simulink model "PID_cascaded_control"  (R2025a)
settings: Solver=FixedStepAuto  StartTime=0.0  StopTime=60  FixedStep=0.01  RelTol=1e-3
InitFcn:
  | parameters
values from neighbouring files (symbols this model uses):
  A = pi*(d/2)^2    (= 0.00321699087728)    [parameters.m]    (also in simulations_code.m = 0.00785398163397; test.m = 0.00785398163397)
  A_cross = 0.090    (= 0.09)    [parameters.m]    (also in simulations_code.m = 0.07; test.m = 0.07)
  C_d = 0.136    [parameters.m]    (also in simulations_code.m = 1; test.m = 1)
  constant_amplitude = 0    [Mission.m]    (also in sensitivity.m)
  d1 = 2    [parameters.m]    (also in simulation_matlab.m = 5; simulations_code.m = 5; test.m = 5)
  disturbance_start_time = 120    [compare_controllers.m]    (also in sensitivity.m = 0)
  F_pos = 0.300 * g + m*g    (= 49.70727)    [parameters.m]    (also in sensitivity.m = 0.300 * g + m_values(i)*g; simulation_matlab.m = 2.94; simulations_code.m = 32.37; test.m = 32.37)
  g = 9.81    [parameters.m]    (also in simulation_matlab.m; simulations_code.m; test.m)
  I_hold = 0    [parameters.m]
  I_move = 1.5    [parameters.m]
  m = 4.567+0.2    (= 4.767)    [parameters.m]    (also in simulation_matlab.m = 3; simulations_code.m = 3; test.m = 3)
  m_a = 0    [parameters.m]    (also in simulation_matlab.m; simulations_code.m = 2.5; test.m = 2.5)
  p = 0.002    [parameters.m]    (also in simulation_matlab.m; simulations_code.m; test.m)
  rho = 1000    [parameters.m]    (also in simulation_matlab.m; simulations_code.m; test.m)
  rpm_max = 150    [parameters.m]
  sine_amplitude = 0    [Mission.m]    (also in sensitivity.m)
  sine_frequency = 0.05    [Mission.m]    (also in sensitivity.m)
  V_supply = 11.1    [parameters.m]
  x_max = V_max / A    (= 0.155424749113)    [parameters.m]    (also in simulations_code.m = 0.0636619772368)
libraries: slpidlib x2
settings Model: Creator=hannasennero  LastModifiedBy=hannasennero
settings SolverCC: ZeroCrossAlgorithm=Adaptive
settings DebuggingCC: IgnoredZcDiagnostic=none

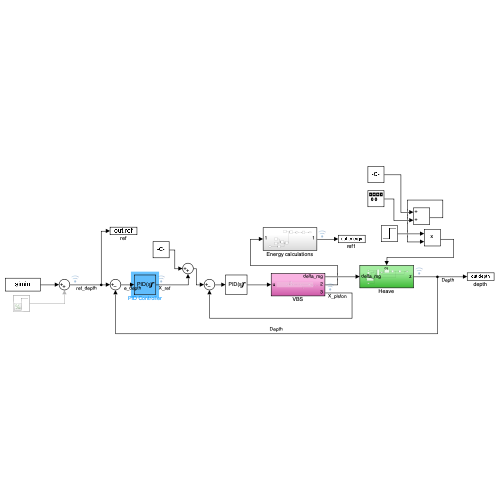
[thumbnail: Simulink's stored preview of the top-level diagram]
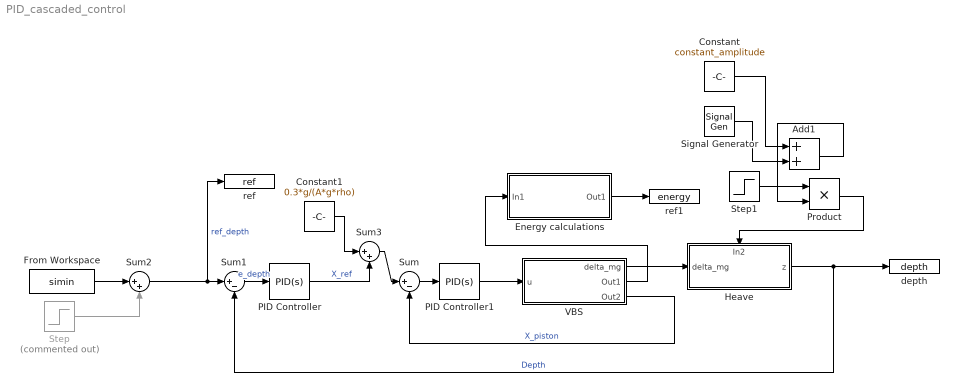
== system PID_cascaded_control ==
  Add1 : Sum
  Constant : Constant  Value=constant_amplitude
  Constant1 : Constant  Value=0.3*g/(A*g*rho)
  Energy calculations : Subsystem
  From Workspace : FromWorkspace  VariableName=simin
  Heave : Subsystem
      settings: PortSchema="{\"entries\":[{\"content\":{\"sides\":[{\"content\":{\"connectorIds\":[\"In1\"]},\"type\":\"ConnectorPlacement.EquallySpacedRectSide\",\"uuid\":\"6f6a1a60-77e6-4781-930b-afddbe975a8d\"},{\"content\":{\"connectorIds\":[\"Out1\"],\"side\":\"RIGHT\"},\"type\":\"ConnectorPlacement.EquallySpacedRectSide\",\"uuid\":\"4976a1b4-b4d2-4f2a-94be-bdc8db839add\"},{\"content\":{\"connectorIds\":[\"In2\"],\"side\":\"TOP\"},\"type\":\"ConnectorPlacement.EquallySpacedRectSide\",\"uuid\":\"504c6e21-38d1-42a8-8b7b-eda0c51b3613\"}]},\"type\":\"ConnectorPlacement.EquallySpacedConnector\",\"uuid\":\"116e8cad-2b5c-4ef7-8338-d893e08918e3\"}],\"packageUris\":[\"http://schema.mathworks.com/mf0/Connector/R2020b\"],\"version\":\"1.0\"}"
  PID Controller : slpidlib/PID Controller  Controller=PID  Form=Parallel  TimeDomain=Continuous-time  UseExternalTs=off  SampleTime=-1  IntegratorMethod=Forward Euler  FilterMethod=Forward Euler  ControllerParametersSource=internal  P=0.1  I=0  UseKiTs=off  D=2  UseExternalDerivativeSource=off  N=10  UseFilter=on  TunerSelectOption=Transfer Function Based (PID Tuner App)  InitialConditionSource=internal  InitialConditionForIntegrator=0  InitialConditionForFilter=0  DifferentiatorICPrevScaledInput=0  ExternalReset=none  TrackingMode=off  Kt=1  LimitOutput=on  SatLimitsSource=internal  UpperSaturationLimit=x_max-0.0003/A  LowerSaturationLimit=-0.0003/A  LinearizeAsGain=off  AntiWindupMode=none  Kb=1  LimitIntegrator=off  UpperIntegratorSaturationLimit=inf  LowerIntegratorSaturationLimit=-inf  POutMin=[]  POutMax=[]  IOutMin=[]  IOutMax=[]  DOutMin=[]  DOutMax=[]  NOutMin=[]  NOutMax=[]  SumOutMin=[]  SumOutMax=[]  SaturationOutMin=[]  SaturationOutMax=[]  PParamMin=[]  PParamMax=[]  IParamMin=[]  IParamMax=[]  DParamMin=[]  DParamMax=[]  NParamMin=[]  NParamMax=[]  KbParamMin=[]  KbParamMax=[]  KtParamMin=[]  KtParamMax=[]  KbOutMin=[]  KbOutMax=[]  KtOutMin=[]  KtOutMax=[]  IntegratorOutMin=[]  IntegratorOutMax=[]  FilterOutMin=[]  FilterOutMax=[]  SumI1OutMin=[]  SumI1OutMax=[]  SumI2OutMin=[]  SumI2OutMax=[]  SumI3OutMin=[]  SumI3OutMax=[]  SumI4OutMin=[]  SumI4OutMax=[]  SumDOutMin=[]  SumDOutMax=[]  DifferentiatorOutMin=[]  DifferentiatorOutMax=[]  FilterDiffOutCoefMin=[]  FilterDiffOutCoefMax=[]  ReciprocalOutMin=[]  ReciprocalOutMax=[]  SumDenOutMin=[]  SumDenOutMax=[]  SumNumOutMin=[]  SumNumOutMax=[]  DivideOutMin=[]  DivideOutMax=[]  UdiffTsProdOutMin=[]  UdiffTsProdOutMax=[]  NTsProdOutMin=[]  NTsProdOutMax=[]  UintegralTsProdOutMin=[]  UintegralTsProdOutMax=[]  UngainTsProdOutMin=[]  UngainTsProdOutMax=[]  ClampingZeroOutDataTypeStr=Inherit: Inherit via back propagation  ClampingZeroOutMin=[]  ClampingZeroOutMax=[]  FilterDenConstantOutDataTypeStr=Inherit: Inherit via back propagation  FilterDenConstantOutMin=[]  FilterDenConstantOutMax=[]  PCopyOutDataTypeStr=Inherit: Inherit via back propagation  PCopyOutMin=[]  PCopyOutMax=[]  NCopyOutDataTypeStr=Inherit: Inherit via back propagation  NCopyOutMin=[]  NCopyOutMax=[]  IntegratorContinuousStateAttributes=''  IntegratorStateMustResolveToSignalObject=off  IntegratorRTWStateStorageClass=Auto  FilterContinuousStateAttributes=''  FilterStateMustResolveToSignalObject=off  FilterRTWStateStorageClass=Auto  ParallelPVariant=InternalParameters  IdealPVariant=Disabled  IVariant=InternalParameters  DVariant=InternalParameters  IntegratorVariant=Continuous  SatVariant=Enabled  AWVariant=Passthrough  PCopyVariant=Disabled  TRVariant=Disabled  FdbkBlocksVariant=Forward  IdealPFdbkVariant=Disabled  SatFdbkVariant=Disabled  DerivativeFilterVariant=ContFilter  NVariant=InternalParameters  NCopyVariant=Disabled  FilterICVariant=InternalICsFilter  IntegratorICVariant=InternalICs  ExternalResetVariant=Disabled  TRSumVariant=Passthrough  SumFdbkVariant=Disabled  SumVariant=Sum_PID  TsampFilterVariant=InternalTs  TsampNgainVariant=Passthrough  TsampIntegralVariant=Disabled_SignalSpec  ExternalSaturationOutDataTypeStr=Inherit: Same as second input  DerivativeSourceVariant=ErrorSignal  PreIntVariant=InternalPreInt
  PID Controller1 : slpidlib/PID Controller  Controller=PID  Form=Parallel  TimeDomain=Continuous-time  UseExternalTs=off  SampleTime=-1  IntegratorMethod=Forward Euler  FilterMethod=Forward Euler  ControllerParametersSource=internal  P=30  I=0  UseKiTs=off  D=0  UseExternalDerivativeSource=off  N=0  UseFilter=on  TunerSelectOption=Transfer Function Based (PID Tuner App)  InitialConditionSource=internal  InitialConditionForIntegrator=0  InitialConditionForFilter=0  DifferentiatorICPrevScaledInput=0  ExternalReset=none  TrackingMode=off  Kt=1  LimitOutput=on  SatLimitsSource=internal  UpperSaturationLimit=1  LowerSaturationLimit=-1  LinearizeAsGain=on  AntiWindupMode=none  Kb=1  LimitIntegrator=off  UpperIntegratorSaturationLimit=inf  LowerIntegratorSaturationLimit=-inf  POutMin=[]  POutMax=[]  IOutMin=[]  IOutMax=[]  DOutMin=[]  DOutMax=[]  NOutMin=[]  NOutMax=[]  SumOutMin=[]  SumOutMax=[]  SaturationOutMin=[]  SaturationOutMax=[]  PParamMin=[]  PParamMax=[]  IParamMin=[]  IParamMax=[]  DParamMin=[]  DParamMax=[]  NParamMin=[]  NParamMax=[]  KbParamMin=[]  KbParamMax=[]  KtParamMin=[]  KtParamMax=[]  KbOutMin=[]  KbOutMax=[]  KtOutMin=[]  KtOutMax=[]  IntegratorOutMin=[]  IntegratorOutMax=[]  FilterOutMin=[]  FilterOutMax=[]  SumI1OutMin=[]  SumI1OutMax=[]  SumI2OutMin=[]  SumI2OutMax=[]  SumI3OutMin=[]  SumI3OutMax=[]  SumI4OutMin=[]  SumI4OutMax=[]  SumDOutMin=[]  SumDOutMax=[]  DifferentiatorOutMin=[]  DifferentiatorOutMax=[]  FilterDiffOutCoefMin=[]  FilterDiffOutCoefMax=[]  ReciprocalOutMin=[]  ReciprocalOutMax=[]  SumDenOutMin=[]  SumDenOutMax=[]  SumNumOutMin=[]  SumNumOutMax=[]  DivideOutMin=[]  DivideOutMax=[]  UdiffTsProdOutMin=[]  UdiffTsProdOutMax=[]  NTsProdOutMin=[]  NTsProdOutMax=[]  UintegralTsProdOutMin=[]  UintegralTsProdOutMax=[]  UngainTsProdOutMin=[]  UngainTsProdOutMax=[]  ClampingZeroOutDataTypeStr=Inherit: Inherit via back propagation  ClampingZeroOutMin=[]  ClampingZeroOutMax=[]  FilterDenConstantOutDataTypeStr=Inherit: Inherit via back propagation  FilterDenConstantOutMin=[]  FilterDenConstantOutMax=[]  PCopyOutDataTypeStr=Inherit: Inherit via back propagation  PCopyOutMin=[]  PCopyOutMax=[]  NCopyOutDataTypeStr=Inherit: Inherit via back propagation  NCopyOutMin=[]  NCopyOutMax=[]  IntegratorContinuousStateAttributes=''  IntegratorStateMustResolveToSignalObject=off  IntegratorRTWStateStorageClass=Auto  FilterContinuousStateAttributes=''  FilterStateMustResolveToSignalObject=off  FilterRTWStateStorageClass=Auto  ParallelPVariant=InternalParameters  IdealPVariant=Disabled  IVariant=InternalParameters  DVariant=InternalParameters  IntegratorVariant=Continuous  SatVariant=Enabled  AWVariant=Passthrough  PCopyVariant=Disabled  TRVariant=Disabled  FdbkBlocksVariant=Forward  IdealPFdbkVariant=Disabled  SatFdbkVariant=Disabled  DerivativeFilterVariant=ContFilter  NVariant=InternalParameters  NCopyVariant=Disabled  FilterICVariant=InternalICsFilter  IntegratorICVariant=InternalICs  ExternalResetVariant=Disabled  TRSumVariant=Passthrough  SumFdbkVariant=Disabled  SumVariant=Sum_PID  TsampFilterVariant=InternalTs  TsampNgainVariant=Passthrough  TsampIntegralVariant=Disabled_SignalSpec  ExternalSaturationOutDataTypeStr=Inherit: Same as second input  DerivativeSourceVariant=ErrorSignal  PreIntVariant=InternalPreInt
  Product : Product
  Signal Generator : SignalGenerator  Amplitude=sine_amplitude  Frequency=sine_frequency  Units=rad/sec
  Step : Step  Commented=on  Time=0.5  SampleTime=0
  Step1 : Step  Time=disturbance_start_time  SampleTime=0
  Sum : Sum  Inputs=|+-
  Sum1 : Sum  Inputs=|+-
  Sum2 : Sum  Inputs=|++
  Sum3 : Sum  Inputs=|++
  VBS : Subsystem
  depth : ToWorkspace  VariableName=depth  SaveFormat=Timeseries  SampleTime=-1
  ref : ToWorkspace  VariableName=ref  SaveFormat=Timeseries  SampleTime=-1
  ref1 : ToWorkspace  VariableName=energy  SaveFormat=Timeseries  SampleTime=-1
  wires:
  Heave/1(z) -> Sum1/2, depth/1  "Depth"
  VBS/1(delta_mg) -> Heave/1(delta_mg)
  From Workspace/1 -> Sum2/1
  VBS/2(Out1) -> Energy calculations/1(In1)
  Energy calculations/1(Out1) -> ref1/1
  Sum1/1 -> PID Controller/1  "e_depth"
  Constant/1 -> Add1/1
  Signal Generator/1 -> Add1/2
  Sum/1 -> PID Controller1/1
  PID Controller1/1 -> VBS/1(u)
  VBS/3(Out2) -> Sum/2  "X_piston"
  Sum2/1 -> ref/1, Sum1/1  "ref_depth"
  Step/1 -> Sum2/2
  Constant1/1 -> Sum3/1
  PID Controller/1 -> Sum3/2  "X_ref"
  Sum3/1 -> Sum/1
  Step1/1 -> Product/1
  Add1/1 -> Product/2
  Product/1 -> Heave/2(In2)

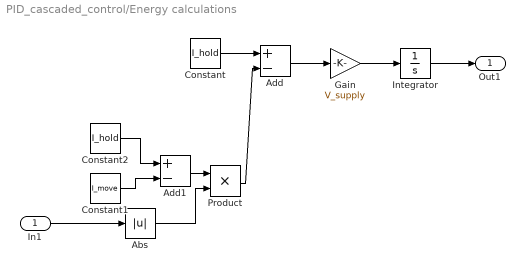
== system PID_cascaded_control/Energy calculations ==
  In1 : Inport
  Abs : Abs  SaturateOnIntegerOverflow=off
  Add : Sum  Inputs=+-
  Add1 : Sum  Inputs=+-
  Constant : Constant  Value=I_hold
  Constant1 : Constant  Value=I_move
  Constant2 : Constant  Value=I_hold
  Gain : Gain  Gain=V_supply
  Integrator : Integrator
  Product : Product
  Out1 : Outport
  wires:
  Constant/1 -> Add/1
  Constant2/1 -> Add1/1
  Constant1/1 -> Add1/2
  Add1/1 -> Product/1
  Product/1 -> Add/2
  Add/1 -> Gain/1
  Gain/1 -> Integrator/1
  Integrator/1 -> Out1/1
  In1/1 -> Abs/1
  Abs/1 -> Product/2

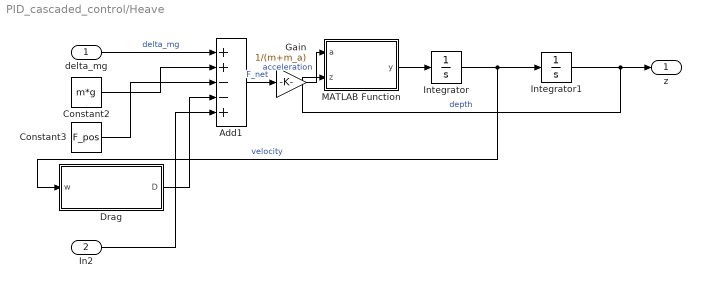
== system PID_cascaded_control/Heave ==
  delta_mg : Inport
  In2 : Inport  Port=2
  Add1 : Sum  Inputs=++--+
  Constant2 : Constant  Value=m*g
  Constant3 : Constant  Value=F_pos
  Drag : Subsystem
  Gain : Gain  Gain=1/(m+m_a)
  Integrator : Integrator  LowerSaturationLimit=0
  Integrator1 : Integrator  LimitOutput=on  LowerSaturationLimit=0
  MATLAB Function : MATLAB Function  TreatAsAtomicUnit=on
  z : Outport
  wires:
  delta_mg/1 -> Add1/1  "delta_mg"
  Constant2/1 -> Add1/2
  Constant3/1 -> Add1/3
  Drag/1(D) -> Add1/4
  Add1/1 -> Gain/1  "F_net"
  Integrator/1 -> Drag/1(w), Integrator1/1  "velocity"
  Integrator1/1 -> MATLAB Function/2(z), z/1  "depth"
  MATLAB Function/1(y) -> Integrator/1
  Gain/1 -> MATLAB Function/1(a)  "acceleration"
  In2/1 -> Add1/5

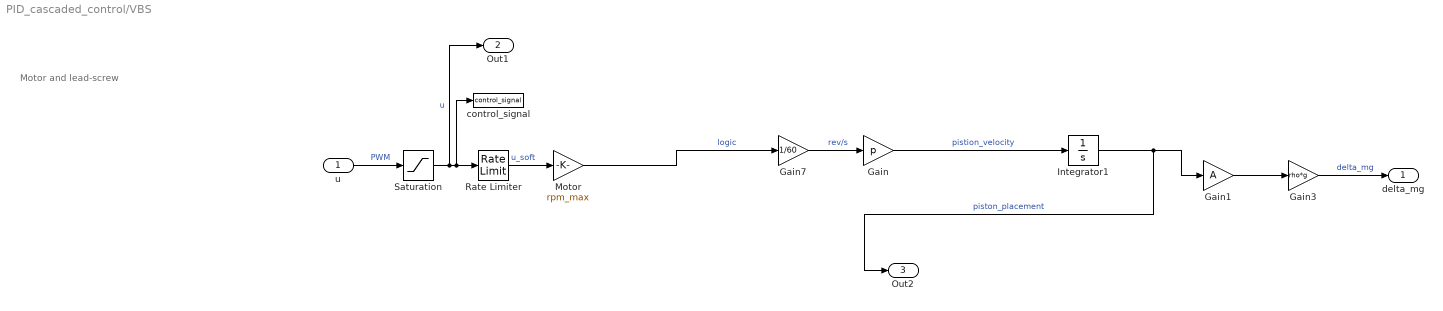
== system PID_cascaded_control/VBS ==
  note: Motor and lead-screw
  u : Inport
  Gain : Gain  Gain=p
  Gain1 : Gain  Gain=A
  Gain3 : Gain  Gain=rho*g
  Gain7 : Gain  Gain=1/60
  Integrator1 : Integrator  InitialCondition=0.3*g/(A*g*rho)  LimitOutput=on  UpperSaturationLimit=x_max  LowerSaturationLimit=0
  Motor : Gain  Gain=rpm_max
  Rate Limiter : RateLimiter  RisingSlewLimit=0.5  FallingSlewLimit=-0.5
  Saturation : Saturate  UpperLimit=1  LowerLimit=-1  LinearizeAsGain=off
  control_signal : ToWorkspace  VariableName=control_signal  SaveFormat=Timeseries  SampleTime=-1
  delta_mg : Outport
  Out1 : Outport  Port=2
  Out2 : Outport  Port=3
  wires:
  u/1 -> Saturation/1  "PWM"
  Gain/1 -> Integrator1/1  "pistion_velocity"
  Integrator1/1 -> Out2/1, Gain1/1  "piston_placement"
  Gain3/1 -> delta_mg/1  "delta_mg"
  Saturation/1 -> Out1/1, Rate Limiter/1, control_signal/1  "u"
  Gain1/1 -> Gain3/1
  Gain7/1 -> Gain/1  "rev/s"
  Motor/1 -> Gain7/1  "logic"
  Rate Limiter/1 -> Motor/1  "u_soft"

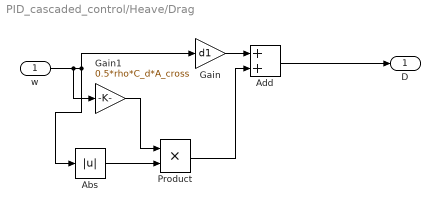
== system PID_cascaded_control/Heave/Drag ==
  w : Inport
  Abs : Abs  SaturateOnIntegerOverflow=off
  Add : Sum
  Gain : Gain  Gain=d1
  Gain1 : Gain  Gain=0.5*rho*C_d*A_cross
  Product : Product
  D : Outport
  wires:
  w/1 -> Gain/1, Abs/1, Gain1/1
  Gain/1 -> Add/1
  Abs/1 -> Product/2
  Gain1/1 -> Product/1
  Product/1 -> Add/2
  Add/1 -> D/1

== matlab function PID_cascaded_control/Heave/MATLAB Function ==
  data: a input; y output; z input
function y = fcn(a,z)
if a<= 0 && z <= 0
    y = 0;
else
    y = a;
end
